simulink model "SimPowerSystems_PWM_Motor_8"  (R2014a)
settings: Solver=FixedStepDiscrete  StartTime=0.0  StopTime=1  RelTol=1e-4
undefined symbols (not defined in the file): level
libraries: powerlib x6, powerlib_extras x1
Description:
  | Copyright 2014 The MathWorks, Inc.
settings Model: Creator=smiller  LastModifiedBy=smiller
settings DataIOCC: SignalLoggingSaveFormat=ModelDataLogs
settings OptimizationCC: ExpressionDepthLimit=2147483647  InitFltsAndDblsToZero=on
settings DebuggingCC: SaveWithParameterizedLinksMsg=none  UnderspecifiedInitializationDetection=Classic  FcnCallInpInsideContextMsg=UseLocalSettings  StateNameClashWarn=warning
settings GRTTargetCC: TargetFcnLib=ansi_tfl_tmw.mat  CombineOutputUpdateFcns=off  GRTInterface=on

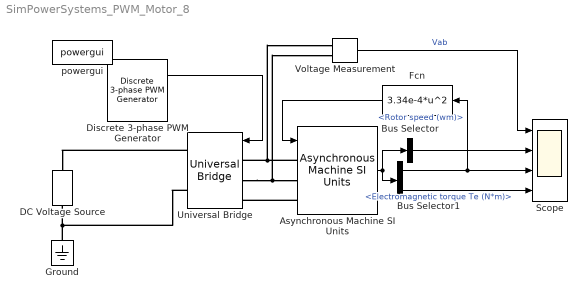
== system SimPowerSystems_PWM_Motor_8 ==
  Asynchronous Machine SI Units : powerlib/Machines/Asynchronous Machine SI Units  PresetModel=No  MechanicalLoad=Torque Tm  ShowDetailedParameters=on  RotorType=Squirrel-cage  ReferenceFrame=Rotor  Units=SI  MeasurementBus=off  NominalParameters=[3*746 220 60]  Stator=[1.115 0.005974]  Rotor=[1.083 0.005974]  Cage1=[ 0.022 0.226/377]  Cage2=[ 0.022 0.226/377]  Lm=0.2037  Mechanical=[0.02 0.005752 2]  PolePairs=2  InitialConditions="[ 1,0   0,0,0   0,0,0 ]"  SimulateSaturation=off  Saturation=[9.9249,19.6672,38.0377,51.3988,69.2824,105.1337,152.5532,214.2421,303.1917;230, 322, 414, 460, 506, 552, 598, 644, 690]  LoadFlowParameters=0  TsPowergui=0  TsBlock=-1  IterativeModel=Forward Euler  Pmec=0
  Bus Selector : BusSelector  OutputSignals=Stator measurements.Stator current is_a (A),Stator measurements.Stator current is_b (A),Stator measurements.Stator current is_c (A)  OutputAsBus=on
  Bus Selector1 : BusSelector  OutputSignals=Mechanical.Rotor speed (wm),Mechanical.Electromagnetic torque Te (N*m)
  DC Voltage Source : powerlib/Electrical Sources/DC Voltage Source  Amplitude=400  Measurements=None
  Discrete 3-phase PWM Generator : powerlib_extras/Discrete  Control Blocks/Discrete 3-phase PWM Generator  ModulatorType=2-level  ModulatorMode=Un-synchronized  nF=18  Fc=18*60  ModulatingSignals=on  m=0.9  Freq=60  Phase=0  Ts=10e-6
  Fcn : Fcn  Expr=3.34e-4*u^2
  Ground : powerlib/Elements/Ground  LConnTagsString=a
  Scope : Scope  NumInputPorts=4
      settings: YMin=-5~-5~-5~-5  YMax=5~5~5~5  SaveName=ASM
  Universal Bridge : powerlib/Power Electronics/Universal Bridge  Arms=3  SnubberResistance=1e5  SnubberCapacitance=inf  Device=IGBT / Diodes  Ron=1e-3  Lon=0  ForwardVoltages="[  0  0  ]"  ForwardVoltage=0  GTOparameters=[ 10e-6 , 20e-6 ]  IGBTparameters=[ 1e-6 , 1e-6 ]  Measurements=None  Measurements_2=None  converterType=Rectifier
  Voltage Measurement : powerlib/Measurements/Voltage Measurement  PhasorSimulation=off  OutputType=Complex  PSBequivalent=0
  powergui : powerlib/powergui  SimulationMode=Discrete  SolverType=Tustin  SampleTime=10e-6  frequency=60  SPID=off  DisableSnubberDevices=off  DisableRonSwitches=off  DisableVfSwitches=off  SwTol=0  Interpol=off  DisplayEquations=off  Ts=0  methode=off  frequencyindice=60  Pbase=100e6  ErrMax=1e-4  Iterations=50  UnitsV=kV  UnitsW=MW  FunctionMessages=off  echomessages=off  HookPort=off  EnableUseOfTLC=off  x0status=blocks  RestoreLinks=warning  ResistiveCurrentMeasurement=off  Frange=[0:2:500]  Ylog=off  Xlog=on  ShowGrid=off  save=off  variable=ZData  structure=ASM  ZoomFFT=on  StartTime=0.7  cycles=2  DisplayStyle=1  fundamental=60  FreqAxis=on  MaxFrequency=5000  frequencyindicesteady=1  RmsSteady=1  display=off
  wires:
  Discrete 3-phase PWM Generator/1 -> Universal Bridge/1
  Asynchronous Machine SI Units/1 -> Bus Selector1/1, Bus Selector/1
  Bus Selector/1 -> Scope/2
  Bus Selector1/1 -> Fcn/1, Scope/3  "<Rotor speed (wm)>"
  Bus Selector1/2 -> Scope/4  "<Electromagnetic torque Te (N*m)>"
  Fcn/1 -> Asynchronous Machine SI Units/1
  Voltage Measurement/1 -> Scope/1  "Vab"
  connections:
  Ground/LConn1 -- DC Voltage Source/LConn1 -- Universal Bridge/RConn2
  Universal Bridge/RConn1 -- DC Voltage Source/RConn1
  Asynchronous Machine SI Units/LConn1 -- Universal Bridge/LConn1 -- Voltage Measurement/LConn1
  Universal Bridge/LConn2 -- Asynchronous Machine SI Units/LConn2 -- Voltage Measurement/LConn2
  Asynchronous Machine SI Units/LConn3 -- Universal Bridge/LConn3
